simulink model "punto_e3"  (R2014a)
settings: Solver=ode45  StartTime=0.0  StopTime=50.0  RelTol=1e-3
values from neighbouring files (symbols this model uses):
  Kc = 1    [es1.m]
  Kr = 1    [es1.m]
  s = tf('s')    [es1.m]
libraries: cstblocks x2, simulink x1
settings Model: Creator=HP  LastModifiedBy=HP

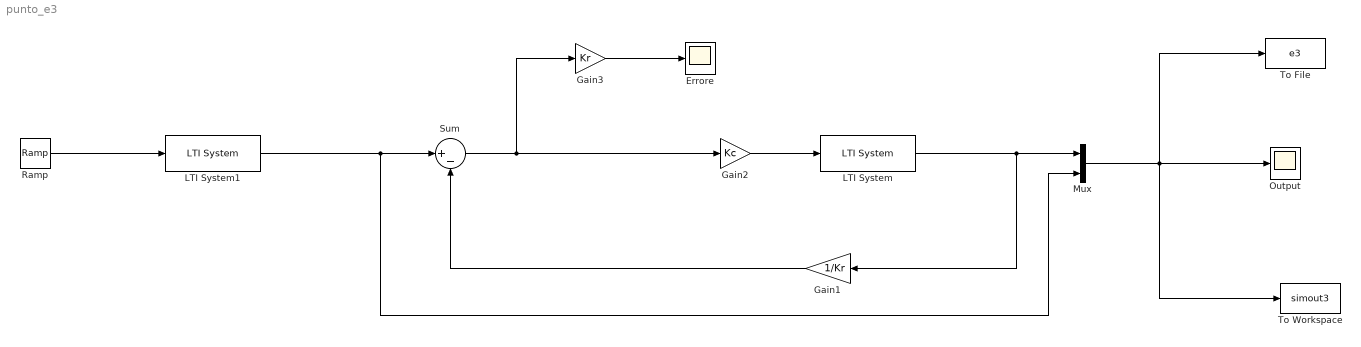
== system punto_e3 ==
  Errore : Scope
  Gain1 : Gain  Gain=1/Kr
  Gain2 : Gain  Gain=Kc
  Gain3 : Gain  Gain=Kr
  LTI System : cstblocks/LTI System  sys=F  IC=[]
  LTI System1 : cstblocks/LTI System  sys=1/s  IC=[]
  Mux : Mux  Inputs=2
  Output : Scope
  Ramp : simulink/Sources/Ramp  slope=1  start=0  X0=0
  Sum : Sum  Inputs=|+-
  To File : ToFile  Filename=e3  MatrixName=output  SaveFormat=Timeseries
  To Workspace : ToWorkspace  VariableName=simout3  SaveFormat=Timeseries  SampleTime=-1
  wires:
  Sum/1 -> Gain3/1, Gain2/1
  Gain1/1 -> Sum/2
  Gain2/1 -> LTI System/1
  LTI System/1 -> Gain1/1, Mux/1
  Mux/1 -> To File/1, To Workspace/1, Output/1
  LTI System1/1 -> Mux/2, Sum/1
  Gain3/1 -> Errore/1
  Ramp/1 -> LTI System1/1
